simulink library "MK_Snowman_Lib"  (R2023b)
settings: Solver=VariableStepAuto  StartTime=0.0  StopTime=10.0  RelTol=1e-3
libraries: simulink x1, $bdroot x1
settings Model: Creator=mluser  LastModifiedBy=FIRSTMentor

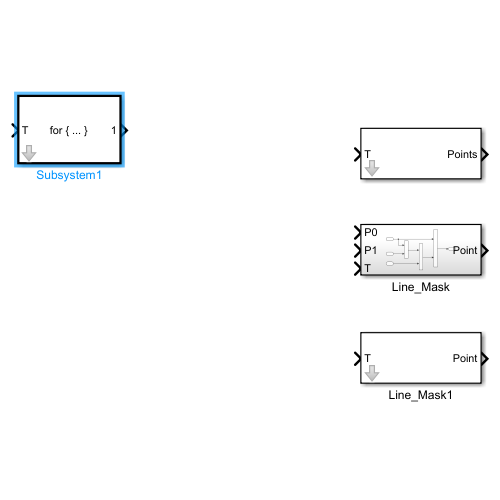
[thumbnail: Simulink's stored preview of the top-level diagram]
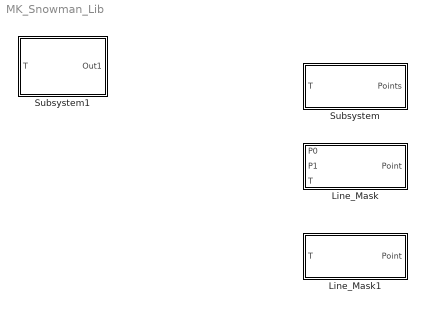
== system MK_Snowman_Lib ==
  Line_Mask : Subsystem
  Line_Mask1 : Subsystem  mask{P0=0, P1=0}
  Subsystem : Subsystem  mask{A=0, B=0, X_Offset=0, Y_Offset=0}
      mask prompts: A "RadiusA"; B "RadiusB"
  Subsystem1 : Subsystem  mask{PointMat=[0, 0 ; 0, 0]}
      mask prompts: PointMat "list of points"

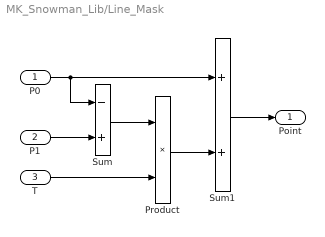
== system MK_Snowman_Lib/Line_Mask ==
  P0 : Inport
  P1 : Inport  Port=2
  T : Inport  Port=3
  Product : Product
  Sum : Sum  Inputs=-+
  Sum1 : Sum
  Point : Outport
  wires:
  P0/1 -> Sum/1, Sum1/1
  P1/1 -> Sum/2
  Sum/1 -> Product/1
  T/1 -> Product/2
  Product/1 -> Sum1/2
  Sum1/1 -> Point/1

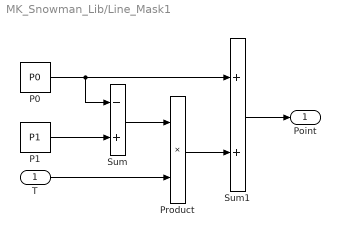
== system MK_Snowman_Lib/Line_Mask1 ==
  T : Inport
  P0 : Constant  Value=P0
  P1 : Constant  Value=P1
  Product : Product
  Sum : Sum  Inputs=-+
  Sum1 : Sum
  Point : Outport
  wires:
  Sum1/1 -> Point/1
  Product/1 -> Sum1/2
  T/1 -> Product/2
  Sum/1 -> Product/1
  P1/1 -> Sum/2
  P0/1 -> Sum1/1, Sum/1

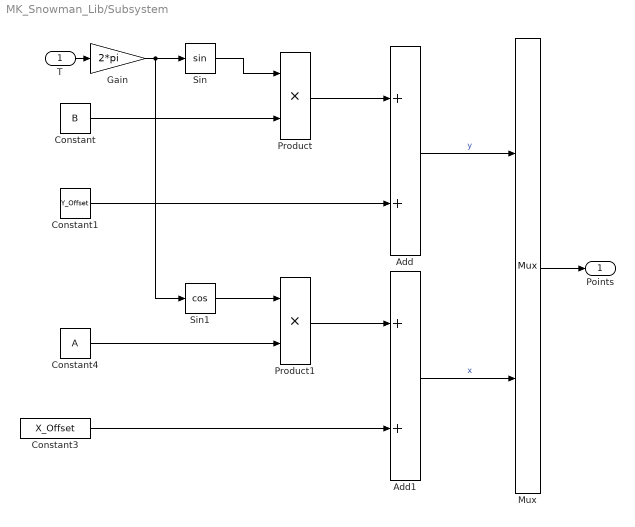
== system MK_Snowman_Lib/Subsystem ==
  T : Inport
  Add : Sum
  Add1 : Sum
  Constant : Constant  Value=B
  Constant1 : Constant  Value=Y_Offset
  Constant3 : Constant  Value=X_Offset
  Constant4 : Constant  Value=A
  Gain : Gain  Gain=2*pi
  Mux : Mux  Inputs=2
  Product : Product
  Product1 : Product
  Sin : Trigonometry
  Sin1 : Trigonometry  Operator=cos
  Points : Outport
  wires:
  Mux/1 -> Points/1
  Product1/1 -> Add1/1
  Constant3/1 -> Add1/2
  Constant4/1 -> Product1/2
  Sin1/1 -> Product1/1
  Gain/1 -> Sin1/1, Sin/1
  Constant1/1 -> Add/2
  Product/1 -> Add/1
  Constant/1 -> Product/2
  Sin/1 -> Product/1
  T/1 -> Gain/1
  Add1/1 -> Mux/2  "x"
  Add/1 -> Mux/1  "y"

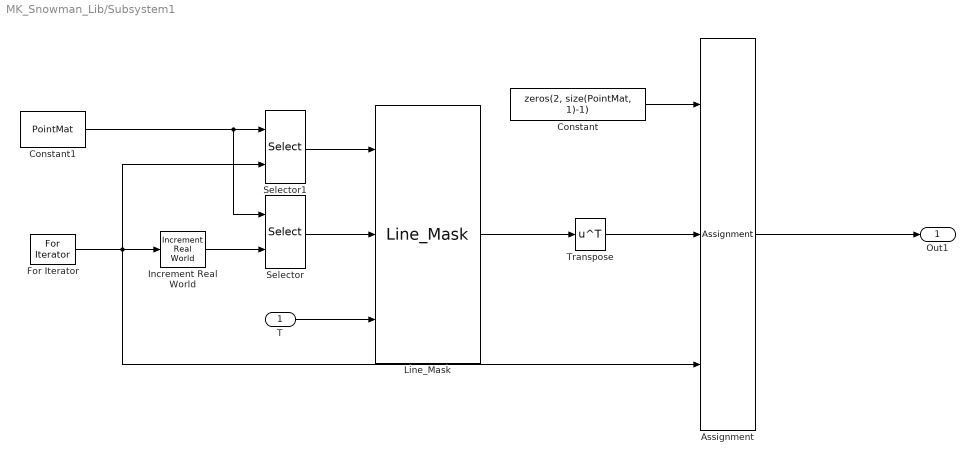
== system MK_Snowman_Lib/Subsystem1 ==
  T : Inport
  Assignment : Assignment  NumberOfDimensions=2  DiagnosticForDimensions=Warning  IndexOptions=Assign all,Index vector (port)  Indices=1,1  OutputSizes=1,1
  Constant : Constant  Value=zeros(2, size(PointMat, 1)-1)  VectorParams1D=off
  Constant1 : Constant  Value=PointMat
  For Iterator : ForIterator  IterationLimit=size(PointMat, 1)-1
  Increment Real World : simulink/Additional Math & Discrete/Additional Math: Increment - Decrement/Increment Real World
  Line_Mask : $bdroot/Line_Mask  SystemSampleTime=-1  VariantActivationTime=update diagram  AllowFlexibleInterface=on  Latency=0  AutoFrameSizeCalculation=off
  Selector : Selector  NumberOfDimensions=2  InputPortWidth=3  IndexOptions=Index vector (port),Select all  Indices=[1 3],1  OutputSizes=1,1
  Selector1 : Selector  NumberOfDimensions=2  InputPortWidth=3  IndexOptions=Index vector (port),Select all  Indices=[1 3],1  OutputSizes=1,1
  Transpose : Math  Operator=transpose
  Out1 : Outport
  wires:
  Selector1/1 -> Line_Mask/1
  For Iterator/1 -> Selector1/2, Increment Real World/1, Assignment/3
  T/1 -> Line_Mask/3
  Increment Real World/1 -> Selector/2
  Constant1/1 -> Selector/1, Selector1/1
  Constant/1 -> Assignment/1
  Selector/1 -> Line_Mask/2
  Assignment/1 -> Out1/1
  Line_Mask/1 -> Transpose/1
  Transpose/1 -> Assignment/2
